simulink model "etc_parent"  (R2022b)
settings: Solver=ode45  StartTime=0.0  StopTime=20.0  RelTol=1e-3
PreLoadFcn:
  | etc_all_data;
values from neighbouring files (symbols this model uses):
  degConv = 180/pi    (= 57.2957795131)    [etc_all_data.m]
  J = 2.4500e-004    (= 0.000245)    [etc_all_data.m]
  Kd = 0.03    [etc_all_data.m]
  Ki = 2    [etc_all_data.m]
  Km = 3.0    (= 3)    [etc_all_data.m]
  Kp = 0.3    [etc_all_data.m]
  Ks = 0.2    [etc_all_data.m]
  theta_eq = pi/6    (= 0.523598775598)    [etc_all_data.m]
  Ts = 0.01    [etc_all_data.m]
Description:
  | This is my help
settings Model: ParamWorkspaceSource=ReferencedWorkspace  Creator=nicholas  LastModifiedBy=bensweet
settings SolverCC: AlgebraicLoopSolver=TrustRegion
settings DataIOCC: LimitDataPoints=on  SaveFormat=Array  ReturnWorkspaceOutputs=off  SignalLoggingName=sigsOut
settings OptimizationCC: ExpressionDepthLimit=2147483647  InitFltsAndDblsToZero=on  LifeSpan=inf
settings DebuggingCC: UnconnectedInputMsg=warning  UnconnectedOutputMsg=warning  UnconnectedLineMsg=warning  PregeneratedLibrarySubsystemCodeDiagnostic=none  SFMachineParentedDataDiag=warning
settings HardwareCC: ProdBitPerPointer=32  ProdBitPerSizeT=32  ProdBitPerPtrDiffT=32  ProdLargestAtomicFloat=None  ProdIntDivRoundTo=Undefined  ProdEndianess=Unspecified  ProdWordSize=32  ProdHWDeviceType=32-bit Generic  TargetIntDivRoundTo=Zero  TargetEndianess=BigEndian  TargetHWDeviceType=Motorola PowerPC
settings ModelReferenceCC: EnableRefExpFcnMdlSchedulingChecks=on  PropagateSignalLabelsOutOfModel=off
settings SFSimCC: SimUseLocalCustomCode=off  SimParseCustomCode=off
settings RTWCC: RTWUseLocalCustomCode=off  DLArmComputeVersion=19.05
settings CodeAppCC: StateflowObjectComments=on
settings GRTTargetCC: TargetFcnLib=ansi_tfl_tmw.mat  TargetLangStandard=C89/C90 (ANSI)  CombineOutputUpdateFcns=off  GRTInterface=on
settings ConfigComp: CovMetricSettings=dw  CovSaveCumulativeToWorkspaceVar=on  CovSaveSingleToWorkspaceVar=on  CovExternalEMLEnable=off  CovSFcnEnable=off

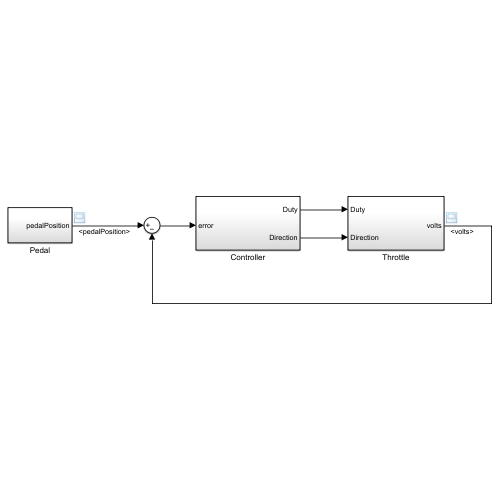
[thumbnail: Simulink's stored preview of the top-level diagram]
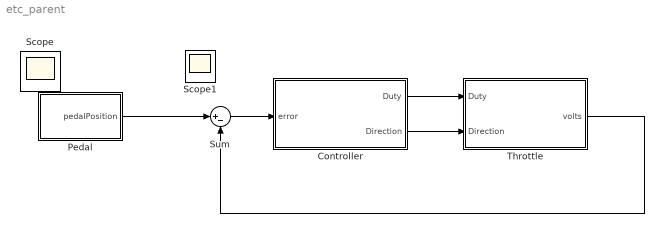
== system etc_parent ==
  Controller : Subsystem
  Pedal : Subsystem
  Sum : Sum  Inputs=|+-
  Throttle : Subsystem
  Scope : Scope
  Scope1 : Scope
  wires:
  Controller/1(Duty) -> Throttle/1(Duty)
  Controller/2(Direction) -> Throttle/2(Direction)
  Pedal/1(pedalPosition) -> Sum/1
  Sum/1 -> Controller/1(error)
  Throttle/1(volts) -> Sum/2

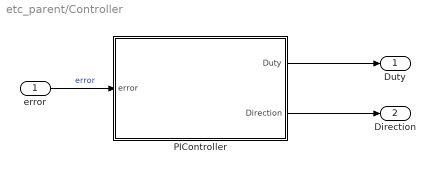
== system etc_parent/Controller ==
  error : Inport
  PIController : Subsystem
  Duty : Outport  VectorParamsAs1DForOutWhenUnconnected=off
  Direction : Outport  Port=2  VectorParamsAs1DForOutWhenUnconnected=off
  wires:
  PIController/2(Direction) -> Direction/1
  PIController/1(Duty) -> Duty/1
  error/1 -> PIController/1(error)  "error"

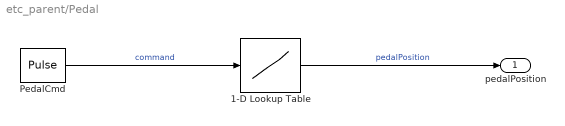
== system etc_parent/Pedal ==
  1-D Lookup Table : Lookup_n-D  NumberOfTableDimensions=1  BreakpointsForDimension1=[0 1]  Table=[0.5 4.5]  RndMeth=Simplest
  PedalCmd : DiscretePulseGenerator  PulseType=Time based  Amplitude=0.9  Period=10  PulseWidth=50  PhaseDelay=2.5
  pedalPosition : Outport  VectorParamsAs1DForOutWhenUnconnected=off
  wires:
  PedalCmd/1 -> 1-D Lookup Table/1  "command"
  1-D Lookup Table/1 -> pedalPosition/1  "pedalPosition"

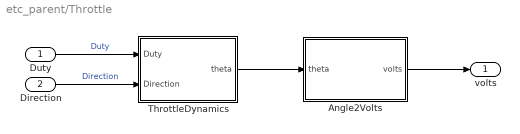
== system etc_parent/Throttle ==
  Duty : Inport
  Direction : Inport  Port=2
  Angle2Volts : Subsystem
  ThrottleDynamics : Subsystem
  volts : Outport  VectorParamsAs1DForOutWhenUnconnected=off
  wires:
  ThrottleDynamics/1(theta) -> Angle2Volts/1(theta)
  Angle2Volts/1(volts) -> volts/1
  Duty/1 -> ThrottleDynamics/1(Duty)  "Duty"
  Direction/1 -> ThrottleDynamics/2(Direction)  "Direction"

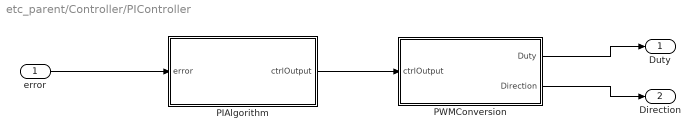
== system etc_parent/Controller/PIController ==
  error : Inport  SampleTime=Ts
  PIAlgorithm : Subsystem
  PWMConversion : Subsystem
  Duty : Outport  VectorParamsAs1DForOutWhenUnconnected=off
  Direction : Outport  Port=2  VectorParamsAs1DForOutWhenUnconnected=off
  wires:
  PIAlgorithm/1(ctrlOutput) -> PWMConversion/1(ctrlOutput)
  PWMConversion/2(Direction) -> Direction/1
  PWMConversion/1(Duty) -> Duty/1
  error/1 -> PIAlgorithm/1(error)

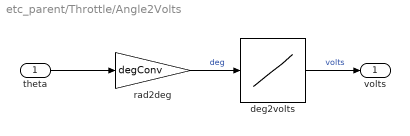
== system etc_parent/Throttle/Angle2Volts ==
  theta : Inport
  deg2volts : Lookup_n-D  NumberOfTableDimensions=1  BreakpointsForDimension1=[0 90]  Table=[0.5 4.5]  RndMeth=Simplest
  rad2deg : Gain  Gain=degConv  SaturateOnIntegerOverflow=on  OutDataTypeStr=Inherit: Same as input  ParamDataTypeStr=Inherit: Same as input
  volts : Outport  VectorParamsAs1DForOutWhenUnconnected=off
  wires:
  rad2deg/1 -> deg2volts/1  "deg"
  deg2volts/1 -> volts/1  "volts"
  theta/1 -> rad2deg/1

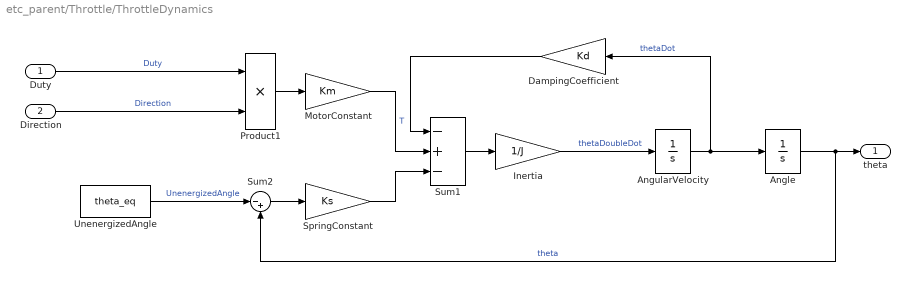
== system etc_parent/Throttle/ThrottleDynamics ==
  Duty : Inport
  Direction : Inport  Port=2
  Angle : Integrator  InitialCondition=pi/6  LimitOutput=on  UpperSaturationLimit=pi/2  LowerSaturationLimit=0
      settings: AttributesFormatString=Initial condition: %<InitialCondition>\n%<LowerSaturationLimit> <= theta <= %<UpperSaturationLimit>
  AngularVelocity : Integrator
      settings: AttributesFormatString=Initial condition: %<InitialCondition>
  DampingCoefficient : Gain  Gain=Kd  SaturateOnIntegerOverflow=on  OutDataTypeStr=Inherit: Same as input  ParamDataTypeStr=Inherit: Same as input
  Inertia : Gain  Gain=1/J  SaturateOnIntegerOverflow=on  OutDataTypeStr=Inherit: Same as input  ParamDataTypeStr=Inherit: Same as input
  MotorConstant : Gain  Gain=Km  SaturateOnIntegerOverflow=on  OutDataTypeStr=Inherit: Same as input  ParamDataTypeStr=Inherit: Same as input
  Product1 : Product  SaturateOnIntegerOverflow=on  OutDataTypeStr=Inherit: Same as first input
  SpringConstant : Gain  Gain=Ks  SaturateOnIntegerOverflow=on  OutDataTypeStr=Inherit: Same as input  ParamDataTypeStr=Inherit: Same as input
  Sum1 : Sum  Inputs=-+-  SaturateOnIntegerOverflow=on
  Sum2 : Sum  Inputs=|-+  SaturateOnIntegerOverflow=on
  UnenergizedAngle : Constant  Value=theta_eq
  theta : Outport  VectorParamsAs1DForOutWhenUnconnected=off
  wires:
  Product1/1 -> MotorConstant/1
  UnenergizedAngle/1 -> Sum2/1  "UnenergizedAngle"
  Sum2/1 -> SpringConstant/1
  Angle/1 -> theta/1, Sum2/2  "theta"
  AngularVelocity/1 -> Angle/1, DampingCoefficient/1  "thetaDot"
  Inertia/1 -> AngularVelocity/1  "thetaDoubleDot"
  Sum1/1 -> Inertia/1
  Duty/1 -> Product1/1  "Duty"
  Direction/1 -> Product1/2  "Direction"
  MotorConstant/1 -> Sum1/2  "T"
  DampingCoefficient/1 -> Sum1/1
  SpringConstant/1 -> Sum1/3

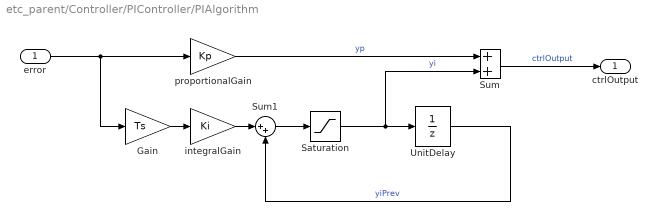
== system etc_parent/Controller/PIController/PIAlgorithm ==
  error : Inport  SampleTime=Ts
      settings: AttributesFormatString=Sample time = %<SampleTime>
  Gain : Gain  Gain=Ts  SaturateOnIntegerOverflow=on  OutDataTypeStr=Inherit: Same as input  ParamDataTypeStr=Inherit: Same as input
  Saturation : Saturate  UpperLimit=1  LowerLimit=-1
      settings: AttributesFormatString=Max: %<UpperLimit>\nMin: %<LowerLimit>
  Sum : Sum  InputSameDT=on  SaturateOnIntegerOverflow=on  OutDataTypeStr=Inherit: Same as first input
  Sum1 : Sum  Inputs=|++  InputSameDT=on  SaturateOnIntegerOverflow=on  OutDataTypeStr=Inherit: Same as first input
  UnitDelay : UnitDelay  SampleTime=Ts  HasFrameUpgradeWarning=on
      settings: AttributesFormatString=yi0 = %<X0>\nSample time = %<SampleTime>
  integralGain : Gain  Gain=Ki  SaturateOnIntegerOverflow=on  OutDataTypeStr=Inherit: Same as input  ParamDataTypeStr=Inherit: Same as input
  proportionalGain : Gain  Gain=Kp  SaturateOnIntegerOverflow=on  OutDataTypeStr=Inherit: Same as input  ParamDataTypeStr=Inherit: Same as input
  ctrlOutput : Outport  VectorParamsAs1DForOutWhenUnconnected=off
  wires:
  Sum/1 -> ctrlOutput/1  "ctrlOutput"
  error/1 -> Gain/1, proportionalGain/1
  Saturation/1 -> Sum/2, UnitDelay/1  "yi"
  Sum1/1 -> Saturation/1
  UnitDelay/1 -> Sum1/2  "yiPrev"
  Gain/1 -> integralGain/1
  integralGain/1 -> Sum1/1
  proportionalGain/1 -> Sum/1  "yp"

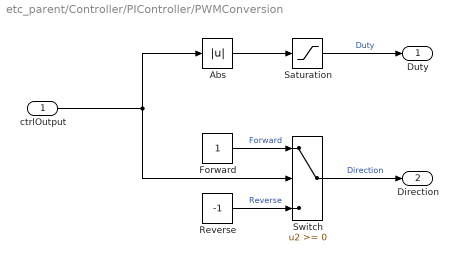
== system etc_parent/Controller/PIController/PWMConversion ==
  ctrlOutput : Inport
  Abs : Abs  SaturateOnIntegerOverflow=off
  Forward : Constant  OutDataTypeStr=double
  Reverse : Constant  Value=-1  OutDataTypeStr=double
  Saturation : Saturate  UpperLimit=1  LowerLimit=0
      settings: AttributesFormatString=%<LowerLimit> < duty < %<UpperLimit>
  Switch : Switch  SaturateOnIntegerOverflow=off  InputSameDT=off
      settings: AttributesFormatString=Criteria: %<Criteria>\nThreshold: %<Threshold>
  Duty : Outport  VectorParamsAs1DForOutWhenUnconnected=off
  Direction : Outport  Port=2  VectorParamsAs1DForOutWhenUnconnected=off
  wires:
  ctrlOutput/1 -> Abs/1, Switch/2
  Forward/1 -> Switch/1  "Forward"
  Reverse/1 -> Switch/3  "Reverse"
  Switch/1 -> Direction/1  "Direction"
  Saturation/1 -> Duty/1  "Duty"
  Abs/1 -> Saturation/1
